simulink model "test_model"  (R2018b)
settings: Solver=FixedStepAuto  StartTime=0.0  StopTime=3  RelTol=1e-3
libraries: TcAdsLib x2
settings Model: Creator=chijiang  LastModifiedBy=chijiang
settings OptimizationCC: LocalBlockOutputs=off
settings RTWCC: SystemTargetFile=TwinCAT.tlc  GenCodeOnly=on  MakeCommand=make_tct  TemplateMakefile=tct_msbuild.tmf  Description=TwinCAT Target  GenerateReport=on  Toolchain=Microsoft Visual C++ 2017 v15.0 | nmake (64-bit Windows)  TargetLang=C++
settings STFCustomTargetCC: TargetLangStandard=C++03 (ISO)  CompOptLevelCompliant=on  MATLABClassNameForMDSCustomization=Simulink.SoftwareTarget.TargetSpecificTriggerConfigurationBase  GRTInterface=on  SystemTargetFile=TwinCAT.tlc

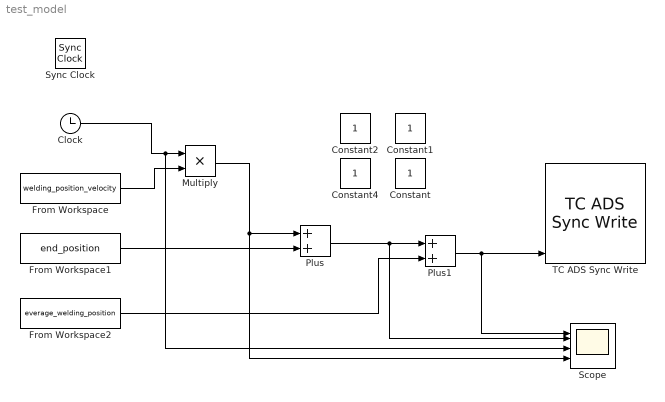
== system test_model ==
  Clock : Clock
  Constant{,1..2,4} (4 alike) : Constant
  From Workspace : FromWorkspace  VariableName=welding_position_velocity  SampleTime=0
  From Workspace1 : FromWorkspace  VariableName=end_position  SampleTime=0
  From Workspace2 : FromWorkspace  VariableName=everage_welding_position  SampleTime=0
  Multiply : Product
  Plus : Sum
  Plus1 : Sum
  Scope : Scope  NumInputPorts=6
  Sync Clock : TcAdsLib/Utilities/Sync Clock  OutputPortSelect=None  InputPortSelect=None
      settings: SourceProductName=Beckhoff TwinCAT ADS Interface
  TC ADS Sync Write : TcAdsLib/Synchronous/TC ADS Sync Write  SampleTime=-1  AbortSimulationOnAdsError=off  WriteDataType=double  WriteDataDim=1  WriteDataColToRowMajor=on  AdsTimeout=1  DirectFeedThrough=off  CreateSignalLabels=on  CodeGenConnectType=DataArea (OutputSrc)
      settings: SourceProductName=Beckhoff TwinCAT ADS Interface
  wires:
  From Workspace1/1 -> Plus/2
  Clock/1 -> Multiply/1, Scope/4
  From Workspace/1 -> Multiply/2
  Multiply/1 -> Scope/6, Plus/1
  Plus/1 -> Scope/2, Plus1/1
  From Workspace2/1 -> Plus1/2
  Plus1/1 -> Scope/1, TC ADS Sync Write/5
